simulink model "untitled"  (R2014b)
settings: Solver=ode45  StartTime=0.0  StopTime=meas.time(end)  RelTol=1e-3
values from neighbouring files (symbols this model uses):
  alpha0 = 1.5568e-6    (= 1.5568e-06)    [InitPar.m]
  alpha1 = 6.1744e-6    (= 6.1744e-06)    [InitPar.m]
  beta0 = Pf/we_idle    (= 16.6666666667)    [InitPar.m]
  eta0 = 0.3676    [InitPar.m]    (also in modelerror2.m = par(1))
  eta1 = -1.3443e-4    (= -0.00013443)    [InitPar.m]    (also in modelerror2.m = par(2))
  eta_gen = 0.7    [InitPar.m]
  gamma0 = 0.5313    [InitPar.m]
  gamma1 = 0.0029    [InitPar.m]
  Hl = 42.5e6    (= 42500000)    [InitPar.m]
  inertia_e = 0.23    [InitPar.m]
  kappa = 1.35    [InitPar.m]
  lambda = 1    [InitPar.m]
  R = 0.01    [IdleSpeedControl.m]    (also in InitPar.m = 287)
  sigma0 = 14.67    [InitPar.m]
  Vc = 2.48e-4    (= 0.000248)    [InitPar.m]
  Vd = 2.48e-3    (= 0.00248)    [InitPar.m]
  Vm = 0.0057    [InitPar.m]    (also in modelerror.m = par; modelerror2.m = par(3); pm_error.m = simulation_parameters)
undefined symbols (not defined in the file or in its folder): meas
settings Model: Creator=kohm  LastModifiedBy=kohm

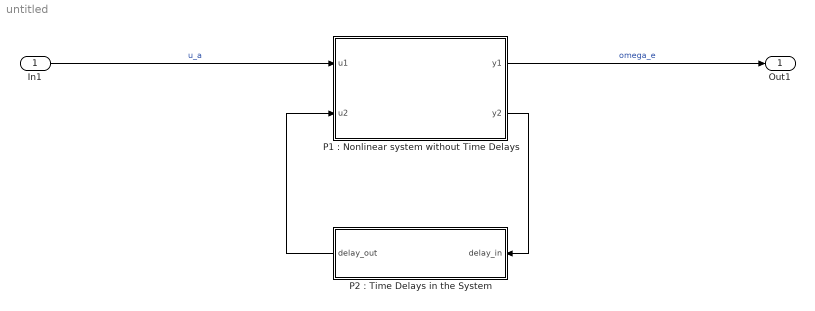
== system untitled ==
  In1 : Inport
  "P1 : Nonlinear system without Time Delays" : Subsystem
  "P2 : Time Delays in the System" : Subsystem
  Out1 : Outport
  wires:
  In1/1 -> "P1 : Nonlinear system without Time Delays"/1(u1)  "u_a"
  "P1 : Nonlinear system without Time Delays"/2(y2) -> "P2 : Time Delays in the System"/1(delay_in)
  "P2 : Time Delays in the System"/1(delay_out) -> "P1 : Nonlinear system without Time Delays"/2(u2)
  "P1 : Nonlinear system without Time Delays"/1(y1) -> Out1/1  "omega_e"

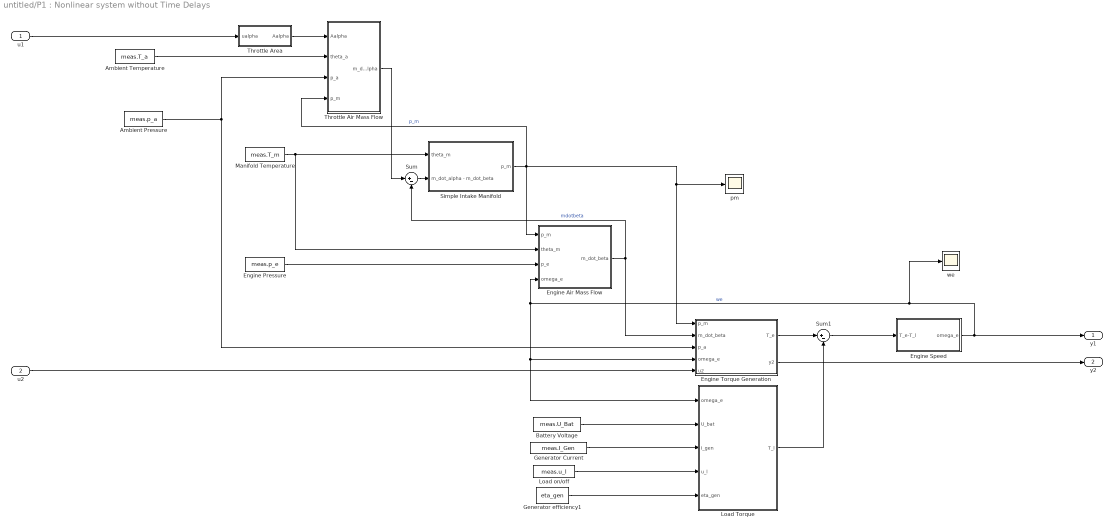
== system untitled/P1 : Nonlinear system without Time Delays ==
  u1 : Inport
  u2 : Inport  Port=2
  Ambient Pressure : FromWorkspace  VariableName=meas.p_a  SampleTime=0
  Ambient Temperature : FromWorkspace  VariableName=meas.T_a  SampleTime=0
  Battery Voltage : FromWorkspace  VariableName=meas.U_Bat  SampleTime=0
  Engine Air Mass Flow : Subsystem
  Engine Pressure : FromWorkspace  VariableName=meas.p_e  SampleTime=0
  Engine Speed : Subsystem
  Engine Torque Generation : Subsystem
  Generator Current : FromWorkspace  VariableName=meas.I_Gen  SampleTime=0
  Generator efficiency1 : Constant  Value=eta_gen
  Load Torque : Subsystem
  Load on/off : FromWorkspace  VariableName=meas.u_l  SampleTime=0
  Manifold Temperature : FromWorkspace  VariableName=meas.T_m  SampleTime=0
  "Simple Intake Manifold " : Subsystem
  Sum : Sum  Inputs=|+-
  Sum1 : Sum  Inputs=|+-
  Throttle Air Mass Flow : Subsystem
  Throttle Area : Subsystem
  pm : Scope
  "we " : Scope
      settings: SaveName=ScopeData2
  y1 : Outport
  y2 : Outport  Port=2
  wires:
  u1/1 -> Throttle Area/1(ualpha)
  Throttle Area/1(Aalpha) -> Throttle Air Mass Flow/1(Aalpha)
  Engine Air Mass Flow/1(m_dot_beta) -> Sum/2, Engine Torque Generation/2(m_dot_beta)  "mdotbeta"
  Sum/1 -> "Simple Intake Manifold "/2(m_dot_alpha - m_dot_beta)
  "Simple Intake Manifold "/1("p_m ") -> Engine Air Mass Flow/1(p_m), pm/1, Engine Torque Generation/1(p_m), Throttle Air Mass Flow/4(p_m)  "p_m"
  Engine Torque Generation/1(T_e) -> Sum1/1
  Load Torque/1(T_l) -> Sum1/2
  Sum1/1 -> Engine Speed/1("T_e-T_l ")
  Engine Speed/1(omega_e) -> y1/1, "we "/1, Engine Air Mass Flow/4(omega_e), Engine Torque Generation/4(omega_e), Load Torque/1(omega_e)  "we"
  Load on/off/1 -> Load Torque/4(u_l)
  Manifold Temperature/1 -> Engine Air Mass Flow/2(theta_m), "Simple Intake Manifold "/1(theta_m)
  Battery Voltage/1 -> Load Torque/2(U_bat)
  Generator Current/1 -> Load Torque/3(I_gen)
  Engine Pressure/1 -> Engine Air Mass Flow/3(p_e)
  Ambient Temperature/1 -> Throttle Air Mass Flow/2(theta_a)
  Ambient Pressure/1 -> Engine Torque Generation/3(p_a), Throttle Air Mass Flow/3(p_a)
  Generator efficiency1/1 -> Load Torque/5(eta_gen)
  Throttle Air Mass Flow/1(m_dot_alpha) -> Sum/1
  Engine Torque Generation/2(y2) -> y2/1
  u2/1 -> Engine Torque Generation/5(u2)

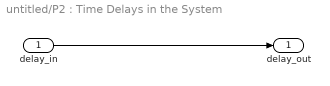
== system untitled/P2 : Time Delays in the System ==
  delay_in : Inport
  delay_out : Outport
  wires:
  delay_in/1 -> delay_out/1

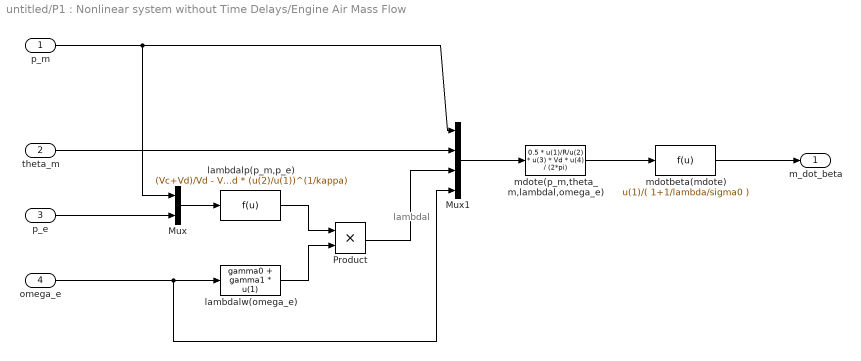
== system untitled/P1 : Nonlinear system without Time Delays/Engine Air Mass Flow ==
  note: lambdal
  p_m : Inport
  theta_m : Inport  Port=2
  p_e : Inport  Port=3
  omega_e : Inport  Port=4
  Mux : Mux  Inputs=2
  Mux1 : Mux
  Product : Product
  lambdalp(p_m,p_e) : Fcn  Expr=(Vc+Vd)/Vd - Vc/Vd * (u(2)/u(1))^(1/kappa)
  lambdalw(omega_e) : Fcn  Expr=gamma0 + gamma1 * u(1)
  mdotbeta(mdote) : Fcn  Expr=u(1)/( 1+1/lambda/sigma0 )
  mdote(p_m,theta_m,lambdal,omega_e) : Fcn  Expr=0.5 * u(1)/R/u(2) * u(3) * Vd * u(4) / (2*pi)
  m_dot_beta : Outport
  wires:
  lambdalw(omega_e)/1 -> Product/2
  lambdalp(p_m,p_e)/1 -> Product/1
  Product/1 -> Mux1/3
  Mux/1 -> lambdalp(p_m,p_e)/1
  p_e/1 -> Mux/2
  p_m/1 -> Mux/1, Mux1/1
  omega_e/1 -> Mux1/4, lambdalw(omega_e)/1
  Mux1/1 -> mdote(p_m,theta_m,lambdal,omega_e)/1
  theta_m/1 -> Mux1/2
  mdote(p_m,theta_m,lambdal,omega_e)/1 -> mdotbeta(mdote)/1
  mdotbeta(mdote)/1 -> m_dot_beta/1

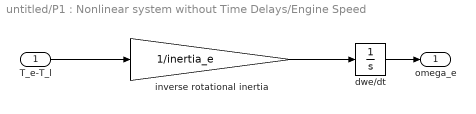
== system untitled/P1 : Nonlinear system without Time Delays/Engine Speed ==
  "T_e-T_l " : Inport
  dwe/dt : Integrator  InitialCondition=meas.omega_e.signals.values(1)  LowerSaturationLimit=0  ContinuousStateAttributes='w_e'
  inverse rotational inertia : Gain  Gain=1/inertia_e
  omega_e : Outport
  wires:
  "T_e-T_l "/1 -> inverse rotational inertia/1
  inverse rotational inertia/1 -> dwe/dt/1
  dwe/dt/1 -> omega_e/1

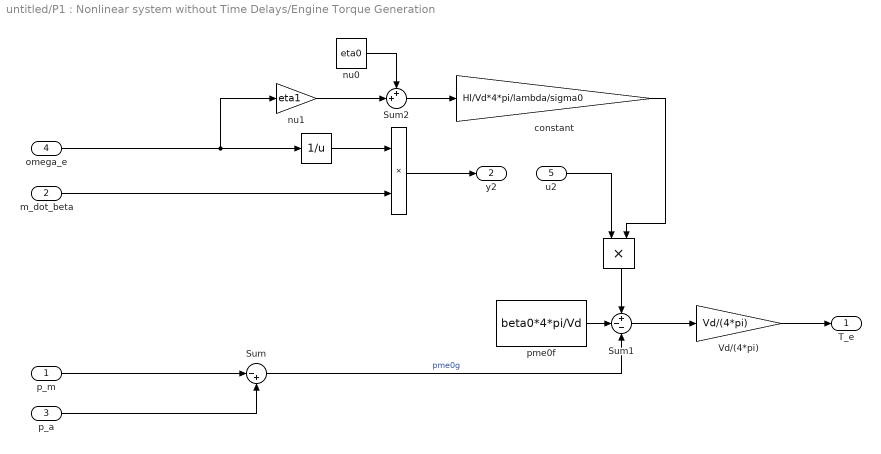
== system untitled/P1 : Nonlinear system without Time Delays/Engine Torque Generation ==
  p_m : Inport
  m_dot_beta : Inport  Port=2
  p_a : Inport  Port=3
  omega_e : Inport  Port=4
  u2 : Inport  Port=5
  " " : Product
  " " : Math  Operator=reciprocal  SaturateOnIntegerOverflow=on
  " " : Product
  Sum : Sum  Inputs=|-+
  Sum1 : Sum  Inputs=+--
  Sum2 : Sum  Inputs=++|
  Vd/(4*pi) : Gain  Gain=Vd/(4*pi)
  constant : Gain  Gain=Hl/Vd*4*pi/lambda/sigma0
  "nu0 " : Constant  Value=eta0
  "nu1 " : Gain  Gain=eta1
  pme0f : Constant  Value=beta0*4*pi/Vd
  T_e : Outport
  y2 : Outport  Port=2
  wires:
  Vd/(4*pi)/1 -> T_e/1
  p_m/1 -> Sum/1
  Sum1/1 -> Vd/(4*pi)/1
  Sum/1 -> Sum1/3  "pme0g"
  pme0f/1 -> Sum1/2
  "nu0 "/1 -> Sum2/1
  "nu1 "/1 -> Sum2/2
  Sum2/1 -> constant/1
  constant/1 -> " "/2
  " "/1 -> Sum1/1
  " "/1 -> " "/1
  m_dot_beta/1 -> " "/2
  " "/1 -> y2/1
  p_a/1 -> Sum/2
  omega_e/1 -> " "/1, "nu1 "/1
  u2/1 -> " "/1

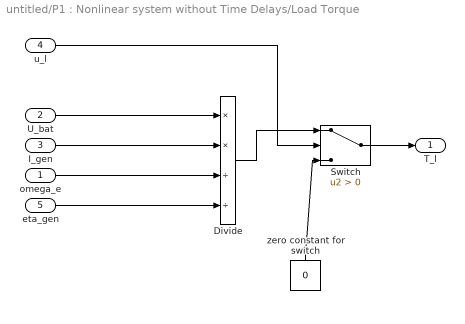
== system untitled/P1 : Nonlinear system without Time Delays/Load Torque ==
  omega_e : Inport
  U_bat : Inport  Port=2
  I_gen : Inport  Port=3
  u_l : Inport  Port=4
  eta_gen : Inport  Port=5
  " zero constant for switch" : Constant  Value=0
  Divide : Product  Inputs=**//
  Switch : Switch  Criteria=u2 > Threshold
  T_l : Outport
  wires:
  U_bat/1 -> Divide/1
  I_gen/1 -> Divide/2
  omega_e/1 -> Divide/3
  eta_gen/1 -> Divide/4
  Divide/1 -> Switch/1
  u_l/1 -> Switch/2
  Switch/1 -> T_l/1
  " zero constant for switch"/1 -> Switch/3

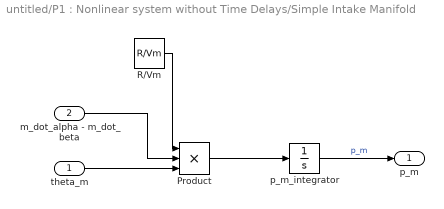
== system untitled/P1 : Nonlinear system without Time Delays/Simple Intake Manifold  ==
  theta_m : Inport
  m_dot_alpha - m_dot_beta : Inport  Port=2
  Product : Product  Inputs=3
  R/Vm : Constant  Value=R/Vm
  p_m_integrator : Integrator  InitialCondition=meas.p_m.signals.values(1)  ContinuousStateAttributes='p_m'
  "p_m " : Outport
  wires:
  p_m_integrator/1 -> "p_m "/1  "p_m"
  Product/1 -> p_m_integrator/1
  theta_m/1 -> Product/3
  m_dot_alpha - m_dot_beta/1 -> Product/2
  R/Vm/1 -> Product/1

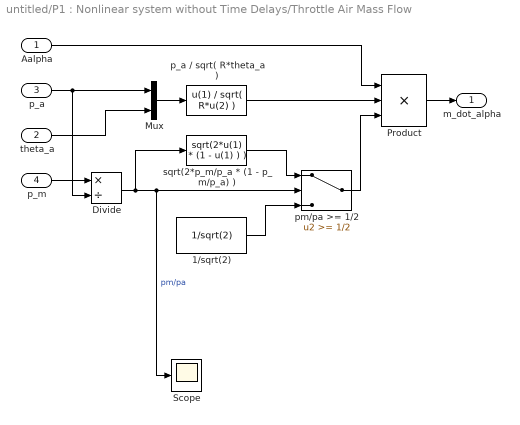
== system untitled/P1 : Nonlinear system without Time Delays/Throttle Air Mass Flow ==
  Aalpha : Inport
  theta_a : Inport  Port=2
  p_a : Inport  Port=3
  p_m : Inport  Port=4
  1/sqrt(2) : Constant  Value=1/sqrt(2)
  Divide : Product  Inputs=*/
  Mux : Mux  Inputs=2
  Product : Product  Inputs=3
  Scope : Scope
      settings: SaveName=ScopeData3
  p_a / sqrt( R*theta_a ) : Fcn  Expr=u(1) / sqrt( R*u(2) )
  pm/pa >= 1/2 : Switch  Threshold=1/2
  sqrt(2*p_m/p_a * (1 - p_m/p_a) ) : Fcn  Expr=sqrt(2*u(1) * (1 - u(1) ) )
  m_dot_alpha : Outport
  wires:
  Mux/1 -> p_a / sqrt( R*theta_a )/1
  theta_a/1 -> Mux/2
  p_a / sqrt( R*theta_a )/1 -> Product/2
  p_a/1 -> Mux/1, Divide/2
  p_m/1 -> Divide/1
  Divide/1 -> Scope/1, pm/pa >= 1/2/2, sqrt(2*p_m/p_a * (1 - p_m/p_a) )/1  "pm/pa"
  1/sqrt(2)/1 -> pm/pa >= 1/2/3
  pm/pa >= 1/2/1 -> Product/3
  sqrt(2*p_m/p_a * (1 - p_m/p_a) )/1 -> pm/pa >= 1/2/1
  Product/1 -> m_dot_alpha/1
  Aalpha/1 -> Product/1

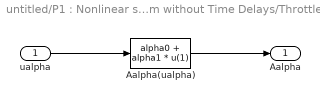
== system untitled/P1 : Nonlinear system without Time Delays/Throttle Area ==
  ualpha : Inport
  Aalpha(ualpha) : Fcn  Expr=alpha0 + alpha1 * u(1)
  Aalpha : Outport
  wires:
  ualpha/1 -> Aalpha(ualpha)/1
  Aalpha(ualpha)/1 -> Aalpha/1
